simulink model "sim_fuelratio"  (R2024a)
settings: Solver=VariableStepAuto  StartTime=0.0  StopTime=10.0  RelTol=1e-3
undefined symbols (not defined in the file): DiscIntNeverNeededParam, dither_amplitude, dither_omega, dt, highpass_filter_discretized, initial_nD, initial_nT, initial_ratio, integral_gain, lowpass_filter_discretized, n_D_dynamics_discretized, n_T_dynamics_discretized, optimizer_gain, proportional_gain, total_density_reference
settings Model: Creator=20181915  LastModifiedBy=20181915

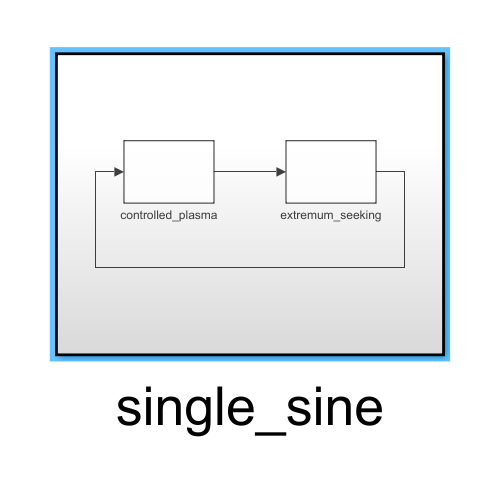
[thumbnail: Simulink's stored preview of the top-level diagram]
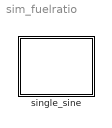
== system sim_fuelratio ==
  single_sine : Subsystem

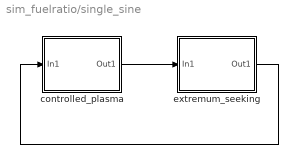
== system sim_fuelratio/single_sine ==
  controlled_plasma : Subsystem
  extremum_seeking : Subsystem
  wires:
  extremum_seeking/1(Out1) -> controlled_plasma/1(In1)
  controlled_plasma/1(Out1) -> extremum_seeking/1(In1)

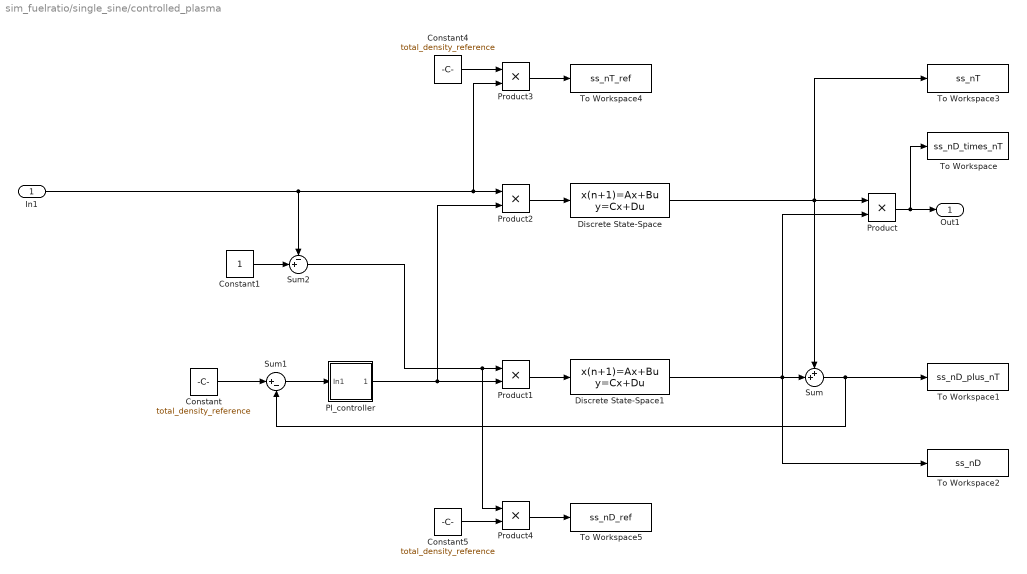
== system sim_fuelratio/single_sine/controlled_plasma ==
  In1 : Inport
  Constant : Constant  Value=total_density_reference
  Constant1 : Constant
  Constant4 : Constant  Value=total_density_reference
  Constant5 : Constant  Value=total_density_reference
  Discrete State-Space : DiscreteStateSpace  A=n_T_dynamics_discretized.A  B=n_T_dynamics_discretized.B  C=n_T_dynamics_discretized.C  D=n_T_dynamics_discretized.D  InitialCondition=initial_nT  SampleTime=-1
  Discrete State-Space1 : DiscreteStateSpace  A=n_D_dynamics_discretized.A  B=n_D_dynamics_discretized.B  C=n_D_dynamics_discretized.C  D=n_D_dynamics_discretized.D  InitialCondition=initial_nD  SampleTime=-1
  PI_controller : Subsystem
  Product{,1..4} (5 alike) : Product
  Sum : Sum  Inputs=++|
  Sum1 : Sum  Inputs=|+-
  Sum2 : Sum  Inputs=-+|
  To Workspace : ToWorkspace  VariableName=ss_nD_times_nT  SampleTime=-1
  To Workspace1 : ToWorkspace  VariableName=ss_nD_plus_nT  SampleTime=-1
  To Workspace2 : ToWorkspace  VariableName=ss_nD  SampleTime=-1
  To Workspace3 : ToWorkspace  VariableName=ss_nT  SampleTime=-1
  To Workspace4 : ToWorkspace  VariableName=ss_nT_ref  SampleTime=-1
  To Workspace5 : ToWorkspace  VariableName=ss_nD_ref  SampleTime=-1
  Out1 : Outport
  wires:
  Product2/1 -> Discrete State-Space/1
  Discrete State-Space/1 -> To Workspace3/1, Product/1, Sum/1
  Constant/1 -> Sum1/1
  In1/1 -> Product3/2, Product2/1, Sum2/1
  Constant1/1 -> Sum2/2
  Discrete State-Space1/1 -> To Workspace2/1, Sum/2, Product/2
  Sum/1 -> To Workspace1/1, Sum1/2
  Product1/1 -> Discrete State-Space1/1
  Product/1 -> To Workspace/1, Out1/1
  PI_controller/1(Out1) -> Product2/2, Product1/2
  Sum1/1 -> PI_controller/1(In1)
  Product3/1 -> To Workspace4/1
  Constant4/1 -> Product3/1
  Sum2/1 -> Product4/1, Product1/1
  Constant5/1 -> Product4/2
  Product4/1 -> To Workspace5/1

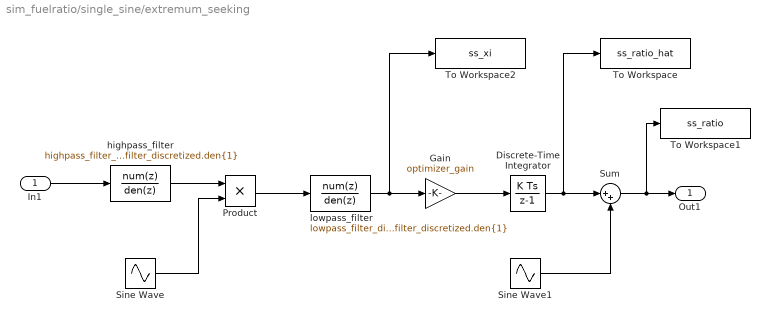
== system sim_fuelratio/single_sine/extremum_seeking ==
  In1 : Inport
  Discrete-Time Integrator : DiscreteIntegrator  InitialCondition=initial_ratio  SampleTime=-1  ICPrevOutput=DiscIntNeverNeededParam  ICPrevScaledInput=DiscIntNeverNeededParam
  Gain : Gain  Gain=optimizer_gain
  Product : Product
  Sine Wave : Sin  Amplitude=2/dither_amplitude  Frequency=dither_omega  SampleTime=dt
  Sine Wave1 : Sin  Amplitude=dither_amplitude  Frequency=dither_omega  SampleTime=dt
  Sum : Sum  Inputs=|++
  To Workspace : ToWorkspace  VariableName=ss_ratio_hat  SampleTime=-1
  To Workspace1 : ToWorkspace  VariableName=ss_ratio  SampleTime=-1
  To Workspace2 : ToWorkspace  VariableName=ss_xi  SampleTime=-1
  highpass_filter : DiscreteTransferFcn  Numerator=highpass_filter_discretized.num{1}  Denominator=highpass_filter_discretized.den{1}
  lowpass_filter : DiscreteTransferFcn  Numerator=lowpass_filter_discretized.num{1}  Denominator=lowpass_filter_discretized.den{1}
  Out1 : Outport
  wires:
  Sine Wave/1 -> Product/2
  highpass_filter/1 -> Product/1
  Discrete-Time Integrator/1 -> To Workspace/1, Sum/1
  In1/1 -> highpass_filter/1
  lowpass_filter/1 -> To Workspace2/1, Gain/1
  Product/1 -> lowpass_filter/1
  Sum/1 -> To Workspace1/1, Out1/1
  Gain/1 -> Discrete-Time Integrator/1
  Sine Wave1/1 -> Sum/2

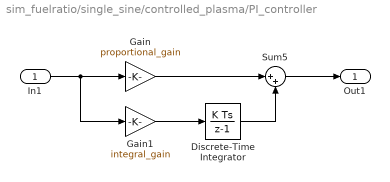
== system sim_fuelratio/single_sine/controlled_plasma/PI_controller ==
  In1 : Inport
  Discrete-Time Integrator : DiscreteIntegrator  SampleTime=-1  ICPrevOutput=DiscIntNeverNeededParam  ICPrevScaledInput=DiscIntNeverNeededParam
  Gain : Gain  Gain=proportional_gain
  Gain1 : Gain  Gain=integral_gain
  Sum5 : Sum  Inputs=|++
  Out1 : Outport
  wires:
  In1/1 -> Gain/1, Gain1/1
  Sum5/1 -> Out1/1
  Discrete-Time Integrator/1 -> Sum5/2
  Gain/1 -> Sum5/1
  Gain1/1 -> Discrete-Time Integrator/1
